simulink model "PWMepitettHidakhozCOSIM"  (R2013b)
settings: Solver=FixedStepDiscrete  SolverMode=SingleTasking  StartTime=0.0  StopTime=260000  FixedStep=0.001  RelTol=1e-3
undefined symbols (not defined in the file or in its folder): A, N
libraries: simulink x2, xbsIndex_r4 x1, JTAGRuntimeCosim_r4 x1
settings Model: Creator=laca  LastModifiedBy=laca

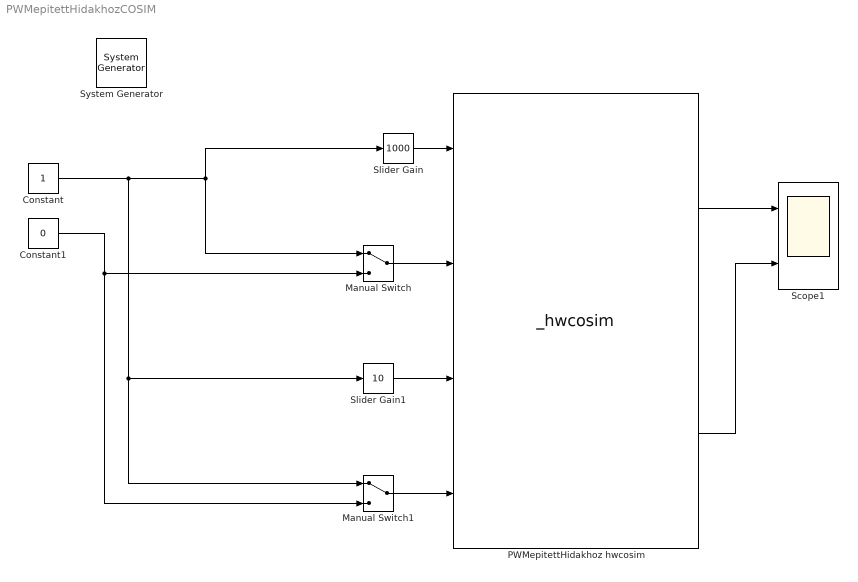
== system PWMepitettHidakhozCOSIM ==
  " System Generator" : xbsIndex_r4/ System Generator  Tag=genX  xilinxfamily=spartan3e  part=xc3s1200e  speed=-4  package=fg320  synthesis_tool=XST  clock_wrapper=Clock Enables  directory=./netlist  proj_type=Project Navigator  Synth_file=XST Defaults  Impl_file=ISE Defaults  testbench=off  simulink_period=1  sysclk_period=20  dcm_input_clock_period=10  incr_netlist=off  trim_vbits=Everywhere in SubSystem  dbl_ovrd=According to Block Masks  core_generation=According to Block Masks  run_coregen=off  deprecated_control=off  eval_field=0  block_type=sysgen
  Constant : Constant
  Constant1 : Constant  Value=0
  Manual Switch : ManualSwitch
  Manual Switch1 : ManualSwitch
  PWMepitettHidakhoz hwcosim : JTAGRuntimeCosim_r4/_hwcosim  clkSrc=Free Running  hasCombinationalPath=off  bitfileName=C:\Diak\gl\SPARTAN3E500K_slave\SystemGenrator\SebessegEsPozicio\netlist\pwmepitetthidakhoz_cw.bit  skipConfig=off  cable=Auto Detect  speed=N/A  cablePort=N/A  cableLocation=Local  shareCable=off  enable_codebug=on  design_xtable=|  engineDll=JTAGCosimEngine.dll  cableWaitTime=10  bscanPos=1  IRLengths=[6,8]  useWaitBox=1  hasBufgmux=on  Scheme=Cosim  useCmdProc=1  hasProc=0  useImpact=0  printLogFile=0  block_type=jtagcosim
      | {
      |   'clkWrapper' => 'pwmepitetthidakhoz_cw',
      |   'clocksGcd' => undef,
      |   'device' => 'xc3s1200e-4fg320',
      |   'ports' => {
      |     'dir' => {
      |       'bd_port_index' => 0,
      |       'direction' => 'in',
      |       'icon_text' => 'DIR',
      |       'period' => 1,
      |       'sim_pause_trigger' => false,
      |       'type' => 'Bool',
      |       'width' => 1,
      |     },
      |     'duty' => {
      |       'bd_port_index' => 1,
      |       'direction' => 'in',
      |       'icon_text' => 'DUTY',
      |       'period' => 1,
      |       'sim_pause_trigger' => false,
      |       'type' => 'UFix_16_0',
      |       'width' => 16,
      |     },
      |     'en' => {
      |       'bd_port_index' => 2,
      |       'direction' => 'in',
      |       'icon_text' => 'En',
      |       'period' => 1,
      |       'sim_pause_trigger' => false,
      |       'type' => 'Bool',
      |       'width' => 1,
      |     },
      |     'speedpwm0' => {
      |       'bd_port_index' => 0,
      |       'direction' => 'out',
      |       'icon_text' => 'SpeedPWM0',
      |       'period' => 1,
      |       'sim_pause_trigger' => false,
      |       'type' => 'UFix_1_0',
      |       'width' => 1,
      |     },
      |     'speedpwm1' => {
      |       'bd_port_index' => 1,
      |       'direction' => 'out',
      |       'icon_text' => 'SpeedPWM1',
      |       'period' => 1,
      |       'sim_pause_trigger' => false,
      |       'type' => 'UFix_1_0',
      |       'width' => 1,
      |     },
      |     'toltesiido' => {
      |       'bd_port_index' => 3,
      |       'direction' => 'in',
      |       'icon_text' => 'TOLTESIIDO',
      |       'period' => 1,
      |       'sim_pause_trigger' => false,
      |       'type' => 'UFix_16_0',
      |       'width' => 16,
      |     },
      |   },
      |   'shared_memories' => {},
      | }
  Scope1 : Scope  NumInputPorts=2
      settings: TickLabels=on  ShowLegends=on  YMin=0~0  YMax=2000~1
  Slider Gain : simulink/Math Operations/Slider Gain  low=0  gain=1000  high=16535
  Slider Gain1 : simulink/Math Operations/Slider Gain  low=0  gain=10  high=1000
  wires:
  Manual Switch/1 -> PWMepitettHidakhoz hwcosim/2
  Slider Gain1/1 -> PWMepitettHidakhoz hwcosim/3
  Manual Switch1/1 -> PWMepitettHidakhoz hwcosim/4
  Slider Gain/1 -> PWMepitettHidakhoz hwcosim/1
  Constant1/1 -> Manual Switch1/2, Manual Switch/2
  Constant/1 -> Manual Switch1/1, Slider Gain1/1, Slider Gain/1, Manual Switch/1
  PWMepitettHidakhoz hwcosim/1 -> Scope1/1
  PWMepitettHidakhoz hwcosim/2 -> Scope1/2
